simulink model "q2x2simETCsup"  (R2025b)
settings: Solver=ode23s  StartTime=0.0  StopTime=15  MaxStep=.1  RelTol=1e-4
values from neighbouring files (symbols this model uses):
  A = zeros(sum(neqs), 4*NK)    [kernelsc.m]    (also in kernelscinv.m; kernelso.m; kernelsoinv.m; q2x2simu.m = zeros(2*xg))
  Ao = A - [P1; P2]*C    [q2x2simu.m]
  B = zeros(2*xg, 1)    [q2x2simu.m]
  Bo = [[P1; P2] + r*B, B]    [q2x2simu.m]
  C = B'    [q2x2simu.m]
  xg = 128    [bounds.m]    (also in q2x2simu.m)
  z0 = [p * v0_ic(x1); v0_ic(x0)]    [histogrametc.m]    (also in q2x2simu.m = [p*v0(x1), v0(x0)]')
  z0hat = 1.5 * z0    [histogrametc.m]    (also in q2x2simu.m = 1.5*z0)
undefined symbols (not defined in the file or in its folder): K1, K2
settings Model: Creator=humaloja  LastModifiedBy=koudohodeflorent

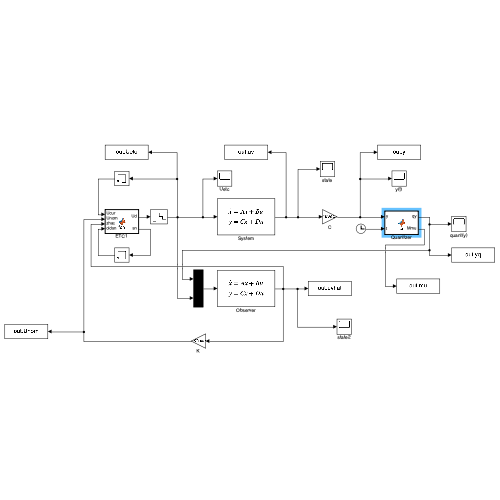
[thumbnail: Simulink's stored preview of the top-level diagram]
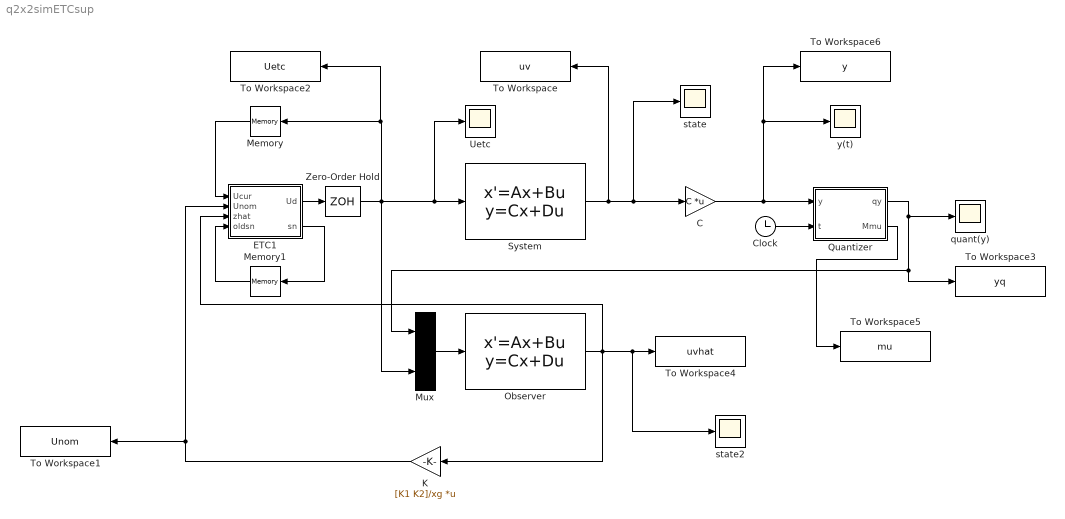
== system q2x2simETCsup ==
  C : Gain  Gain=C  Multiplication=Matrix(K*u) (u vector)
  Clock : Clock
  ETC1 : MATLAB Function  TreatAsAtomicUnit=on
  K : Gain  Gain=[K1 K2]/xg  Multiplication=Matrix(K*u) (u vector)
  Memory : Memory
  Memory1 : Memory
  Mux : Mux  Inputs=2
  Observer : StateSpace  A=Ao  B=Bo  C=eye(2*xg)  D=zeros(2*xg,2)  InitialCondition=z0hat
  Quantizer : MATLAB Function  TreatAsAtomicUnit=on
  System : StateSpace  A=A  B=B  C=eye(2*xg)  D=zeros(2*xg,1)  InitialCondition=z0
  To Workspace : ToWorkspace  VariableName=uv  SaveFormat=Timeseries  SampleTime=-1
  To Workspace1 : ToWorkspace  VariableName=Unom  SaveFormat=Timeseries  SampleTime=-1
  To Workspace2 : ToWorkspace  VariableName=Uetc  SaveFormat=Timeseries  SampleTime=-1
  To Workspace3 : ToWorkspace  VariableName=yq  SaveFormat=Timeseries  SampleTime=-1
  To Workspace4 : ToWorkspace  VariableName=uvhat  SaveFormat=Timeseries  SampleTime=-1
  To Workspace5 : ToWorkspace  VariableName=mu  SaveFormat=Timeseries  SampleTime=-1
  To Workspace6 : ToWorkspace  VariableName=y  SaveFormat=Timeseries  SampleTime=-1
  Uetc : Scope
      settings: ActiveDisplayYMinimum=-18.41524  ActiveDisplayYMaximum=11.25796
  Zero-Order Hold : ZeroOrderHold  SampleTime=-1
  quant(y) : Scope
      settings: ActiveDisplayYMinimum=-10.5  ActiveDisplayYMaximum=4.5  DataLoggingVariableName=ScopeData2
  state : Scope
      settings: ActiveDisplayYMinimum=-5.0111601734068E+8  ActiveDisplayYMaximum=5.567956859341E+7  DataLoggingVariableName=ScopeData4
  state2 : Scope
      settings: ActiveDisplayYMinimum=-20.70698  ActiveDisplayYMaximum=18.96744
  y(t) : Scope
      settings: ActiveDisplayYMinimum=-11.52754  ActiveDisplayYMaximum=6.14184
  wires:
  Mux/1 -> Observer/1
  System/1 -> To Workspace/1, state/1, C/1
  Quantizer/1(qy) -> quant(y)/1, To Workspace3/1, Mux/1
  Clock/1 -> Quantizer/2(t)
  Observer/1 -> K/1, ETC1/3(zhat), state2/1, To Workspace4/1
  Zero-Order Hold/1 -> Mux/2, To Workspace2/1, Memory/1, Uetc/1, System/1
  C/1 -> To Workspace6/1, y(t)/1, Quantizer/1(y)
  Quantizer/2(Mmu) -> To Workspace5/1
  K/1 -> ETC1/2(Unom), To Workspace1/1
  ETC1/2(sn) -> Memory1/1
  Memory1/1 -> ETC1/4(oldsn)
  ETC1/1(Ud) -> Zero-Order Hold/1
  Memory/1 -> ETC1/1(Ucur)

== matlab function q2x2simETCsup/Quantizer ==
  data: y input; qy output; t input; Mmu output
function [qy, Mmu] = fcn(y,t)
% parameters
M = 3; Delta = M/10;
mu0 =5; Omega =.6; T = 2;

% mu
mu = mu0*Omega^floor(t/T);
Mmu = M*mu;

% quantizer
if y/mu > M
  qy = M;
elseif y/mu < -M
  qy = -M;
else
  qy = Delta*floor(y/(mu*Delta) + 0.5);
end
% multiply output by mu
qy = mu*qy;

% FOR TESTING: disable quantization by just returning y
%qy = y;
end

== matlab function q2x2simETCsup/ETC1 ==
  data: Ucur input; Unom input; Ud output; zhat input; oldsn input; sn output
function [Ud,sn] = fcn(Ucur,Unom,zhat,oldsn)
% parameters
Cetm = 0.14; 

% split zhat to uhat and vhat
xg = numel(zhat)/2;

sn = max(oldsn,norm(zhat(1:xg),inf) + norm(zhat(xg+1:2*xg),inf));

if abs(Unom - Ucur) > Cetm*sn
  Ud = Unom;
  sn = norm(zhat(1:xg),inf) + norm(zhat(xg+1:2*xg),inf);
else
  Ud = Ucur;
end

% FOR TESTING: disable event-triggering by just returning Unom
% Ud = Unom;
end
